simulink model "AlvaroGaona_08b"  (R2025b)
settings: Solver=VariableStepAuto  StartTime=0.0  StopTime=10.0  RelTol=1e-3
InitFcn:
  | numero = 8;
  | rng(numero);
  | valor = rand;
  | 
  | M = 1 + valor/2;
  | m = 0.2 * (1 + valor);
  | b = 0.1 * (1 + valor);
  | l = 0.3 * (1.5 - valor/2);
  | g = 9.81;
  | 
  | A = [0, 1, 0, 0;
  | 0, -b/M, -m*g/M, 0;
  | 0, 0, 0, 1;
  | 0, b/(M*l), (M+m)*g/(M*l), 0];
  | 
  | B_ss = [0; 1/M; 0; -1/(M*l)];
  | C_ss = eye(4);
  | D_ss = zeros(4,1);
  | 
  | T = 0.02;
  | sys_d = c2d(ss(A, B_ss, C_ss, D_ss), T, 'zoh');
  | Ad = sys_d.A;
  | Bd = sys_d.B;
  | 
  | Q = diag([100, 80, 10, 1]);
  | R = 10;
  | [K, ~, ~] = dlqr(Ad, Bd, Q, R);
  | 
  | x0 = [0; 0; 0; 0];
  | X_F = [0.5; 0; 0; 0];
undefined symbols (not defined in the file or in its folder): K
settings Model: Creator=alvaro  LastModifiedBy=alvaro

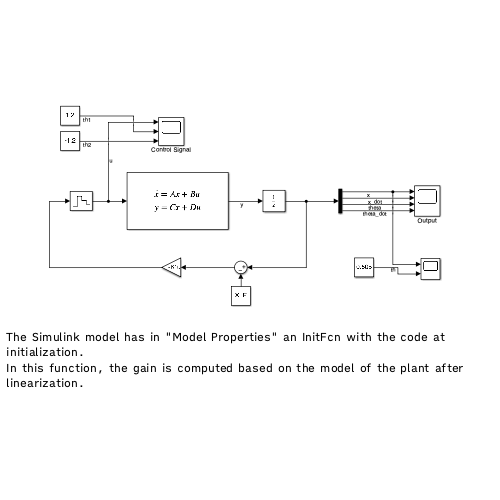
[thumbnail: Simulink's stored preview of the top-level diagram]
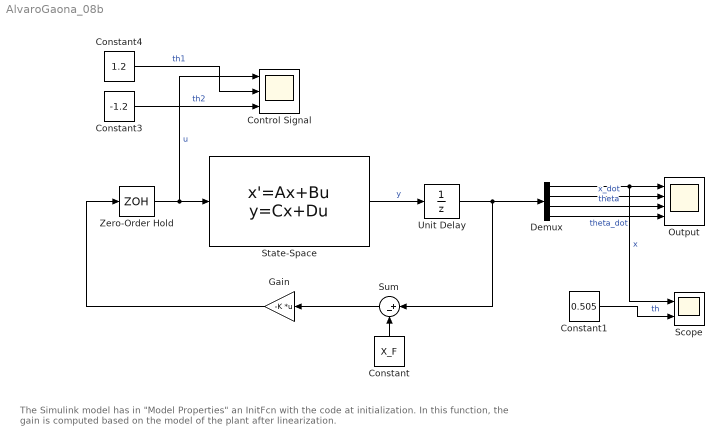
== system AlvaroGaona_08b ==
  note: The Simulink model has in "Model Properties" an InitFcn with the code at initialization.
      | In this function, the gain is computed based on the model of the plant after linearization.
  Constant : Constant  Value=X_F
  Constant1 : Constant  Value=0.505
  Constant3 : Constant  Value=-1.2
  Constant4 : Constant  Value=1.2
  Control Signal : Scope  NumInputPorts=3
      settings: ActiveDisplayYMinimum=-1.4999999999999998  ActiveDisplayYMaximum=1.4999999999999998  DataLoggingVariableName=ScopeData2
  Demux : Demux
  Gain : Gain  Gain=-K  Multiplication=Matrix(K*u)
  Output : Scope  NumInputPorts=4
      settings: ActiveDisplayYMinimum=-0.14133219462899999  ActiveDisplayYMaximum=0.57177665773476849
  Scope : Scope  NumInputPorts=2
      settings: ActiveDisplayYMinimum=0.49642917743445786  ActiveDisplayYMaximum=0.50617397795615793
  State-Space : StateSpace  A=A  B=B_ss  C=C_ss  D=D_ss  InitialCondition=x0
  Sum : Sum  Inputs=|+-
  Unit Delay : UnitDelay  InitialCondition=x0  SampleTime=T  HasFrameUpgradeWarning=on
  Zero-Order Hold : ZeroOrderHold  SampleTime=T
  wires:
  State-Space/1 -> Unit Delay/1  "y"
  Unit Delay/1 -> Sum/1, Demux/1
  Zero-Order Hold/1 -> Control Signal/1, State-Space/1  "u"
  Gain/1 -> Zero-Order Hold/1
  Demux/1 -> Scope/1, Output/1  "x"
  Demux/2 -> Output/2  "x_dot"
  Demux/3 -> Output/3  "theta"
  Demux/4 -> Output/4  "theta_dot"
  Sum/1 -> Gain/1
  Constant/1 -> Sum/2
  Constant1/1 -> Scope/2  "th"
  Constant4/1 -> Control Signal/2  "th1"
  Constant3/1 -> Control Signal/3  "th2"
